simulink model "DDCU_wxt_v02_forA_LabviewV01"  (R2014a)
settings: Solver=FixedStepDiscrete  StartTime=0.0  StopTime=50  FixedStep=0.0005  RelTol=1e-3
InitFcn:
  | Veh_Par_wxt
values from neighbouring files (symbols this model uses):
  ag_thr = 0.4*g    (= 3.924)    [Veh_Par_wxt.m]
  B = 2.25    [Veh_Par_wxt.m]
  bra_pre_em = 12    [Veh_Par_wxt.m]
  bra_pre_gz2 = 12/3    (= 4)    [Veh_Par_wxt.m]
  bra_pre_gz34 = 12/3    (= 4)    [Veh_Par_wxt.m]
  bra_pre_yd = 12/2    (= 6)    [Veh_Par_wxt.m]
  brakepre_dem_data = [0 1 2 3 4 5 6 7 8 9 10 11 12]    [Veh_Par_wxt.m]
  brakeTrq_dem_data = [0 218.198 436.396 654.594 872.792 1090.99 1309.188 1527.386 1745.584 1963.782 2181.98 2400.178 2618.376]    [Veh_Par_wxt.m]
  bratrq_max = 4*2618.376    (= 10473.504)    [Veh_Par_wxt.m]
  eff_tran = 0.75    [Veh_Par_wxt.m]
  G = Mass*g    (= 36297)    [Veh_Par_wxt.m]
  kd1 = 1    [Veh_Par_wxt.m]
  kd2 = 1    [Veh_Par_wxt.m]
  kd3 = 1    [Veh_Par_wxt.m]
  ki1 = 1    [Veh_Par_wxt.m]
  ki2 = 1    [Veh_Par_wxt.m]
  ki3 = 1    [Veh_Par_wxt.m]
  kp1 = 1    [Veh_Par_wxt.m]
  kp2 = 1    [Veh_Par_wxt.m]
  kp3 = 1    [Veh_Par_wxt.m]
  L = 3.12    [Veh_Par_wxt.m]
  premax = 12    [Veh_Par_wxt.m]
  Radius = 0.20    (= 0.2)    [Veh_Par_wxt.m]
  s_opt_yi_add = 0.05    [Veh_Par_wxt.m]
  s_opt_zhuan_add = 0.05    [Veh_Par_wxt.m]
  spd_map_mot = [0 100 200 300 360 400 500 600 700 800 900]*tras_ratio    [Veh_Par_wxt.m]
  spdmax = 900*tras_ratio    (= 5580)    [Veh_Par_wxt.m]
  speed_thr_park = 5/3.6/Radius*30/pi    (= 66.3145596216)    [Veh_Par_wxt.m]
  tras_ratio = 6.2    [Veh_Par_wxt.m]
  trq_map_mot = [1200 1200 1200 1200 1200 1080 864 720 617 540 480]/tras_ratio    [Veh_Par_wxt.m]
  trqmax = 80    [Veh_Par_wxt.m]
  v_thr1_b = 5    [Veh_Par_wxt.m]
  v_thr2_b = 20    [Veh_Par_wxt.m]
  v_thr_park = 5    [Veh_Par_wxt.m]
undefined symbols (not defined in the file or in its folder): DiscIntNeverNeededParam
libraries: simulink x169, ec5744lib x9
(part 7 of 13)

== system DDCU_wxt_v02_forA_LabviewV01/MainControl/mode_control/forward/forward/Brake/rr ==
  speed_act_rr : Inport
  v_act : Inport  Port=2
  Add : Sum
  Constant : Constant  Value=eps
  Divide : Product  Inputs=*/
  Gain : Gain  Gain=pi/30
  Gain1 : Gain  Gain=Radius
  Gain2 : Gain  Gain=1/3.6
  Subtract : Sum  Inputs=+-
  s_act_rr : Outport
  wires:
  speed_act_rr/1 -> Gain/1
  Gain/1 -> Gain1/1
  v_act/1 -> Gain2/1
  Subtract/1 -> Divide/1
  Constant/1 -> Add/2
  Add/1 -> Divide/2
  Divide/1 -> s_act_rr/1
  Gain2/1 -> Add/1, Subtract/1
  Gain1/1 -> Subtract/2

== system DDCU_wxt_v02_forA_LabviewV01/MainControl/mode_control/forward/forward/Drive/容错控制 ==
  trq_dem_l : Inport
  trq_dem_r : Inport  Port=2
  trqlim_lf : Inport  Port=3
  trqlim_lr : Inport  Port=4
  trqlim_rf : Inport  Port=5
  trqlim_rr : Inport  Port=6
  guzhang_lf : Inport  Port=7
  guzhang_lr : Inport  Port=8
  guzhang_rf : Inport  Port=9
  guzhang_rr : Inport  Port=10
  Add : Sum
  Add1 : Sum
  Constant : Constant  Value=bra_pre_gz2
  Constant1 : Constant  Value=bra_pre_gz34
  MATLAB Function : MATLAB Function  TreatAsAtomicUnit=on
  Mux : Mux  Inputs=2
  Scope{,1..16} (17 alike) : Scope
      Scope settings: SaveName=ScopeData25
      Scope1 settings: SaveName=ScopeData26
      Scope10 settings: SaveName=ScopeData35
      Scope11 settings: SaveName=ScopeData36
      Scope12 settings: SaveName=ScopeData37
      Scope13 settings: SaveName=ScopeData38
      Scope14 settings: SaveName=ScopeData39
      Scope15 settings: SaveName=ScopeData40
      Scope16 settings: SaveName=ScopeData41
      Scope2 settings: SaveName=ScopeData27
      Scope3 settings: SaveName=ScopeData28
      Scope4 settings: SaveName=ScopeData29
      Scope5 settings: SaveName=ScopeData30
      Scope6 settings: SaveName=ScopeData31
      Scope7 settings: SaveName=ScopeData32
      Scope8 settings: SaveName=ScopeData33
      Scope9 settings: SaveName=ScopeData34
  Subtract : Sum  Inputs=+-
  To Workspace1 : ToWorkspace  VariableName=simout1  SaveFormat=Timeseries  SampleTime=-1
  To Workspace2 : ToWorkspace  VariableName=simout  SaveFormat=Timeseries  SampleTime=-1
  To Workspace3 : ToWorkspace  VariableName=simout2  SaveFormat=Timeseries  SampleTime=-1
  To Workspace4 : ToWorkspace  VariableName=simout3  SaveFormat=Timeseries  SampleTime=-1
  To Workspace5 : ToWorkspace  VariableName=simout4  SaveFormat=Timeseries  SampleTime=-1
  trq_dem_lf : Outport
  trq_dem_lr : Outport  Port=2
  trq_dem_rf : Outport  Port=3
  trq_dem_rr : Outport  Port=4
  bra_pre_l : Outport  Port=5
  bra_pre_r : Outport  Port=6
  wires:
  guzhang_lr/1 -> To Workspace3/1, MATLAB Function/8(guzhang_lr), Scope14/1
  guzhang_rf/1 -> Scope15/1, To Workspace4/1, MATLAB Function/9(guzhang_rf)
  guzhang_rr/1 -> Scope16/1, To Workspace5/1, MATLAB Function/10(guzhang_rr)
  guzhang_lf/1 -> To Workspace2/1, Scope13/1, MATLAB Function/7(guzhang_lf)
  trq_dem_r/1 -> Scope9/1, MATLAB Function/2(trq_dem_r)
  trqlim_lr/1 -> MATLAB Function/4(trqlim_lr)
  trq_dem_l/1 -> Scope8/1, MATLAB Function/1(trq_dem_l)
  trqlim_rf/1 -> Scope10/1, MATLAB Function/5(trqlim_rf)
  trqlim_rr/1 -> Scope12/1, MATLAB Function/6(trqlim_rr)
  trqlim_lf/1 -> MATLAB Function/3(trqlim_lf)
  MATLAB Function/1(trq_dem_lf) -> Scope/1, Add/1, trq_dem_lf/1
  MATLAB Function/2(trq_dem_lr) -> Scope1/1, Add/2, trq_dem_lr/1
  MATLAB Function/3(trq_dem_rf) -> Scope2/1, Add1/1, trq_dem_rf/1
  MATLAB Function/4(trq_dem_rr) -> Scope3/1, Add1/2, trq_dem_rr/1
  MATLAB Function/5(bra_pre_l) -> Scope4/1, bra_pre_l/1
  MATLAB Function/6(bra_pre_r) -> Scope5/1, bra_pre_r/1
  Constant/1 -> MATLAB Function/11(bra_pre_gz2)
  Constant1/1 -> MATLAB Function/12(bra_pre_gz34)
  Add/1 -> Mux/1, Subtract/1
  Add1/1 -> Mux/2, Subtract/2
  Subtract/1 -> Scope6/1
  Mux/1 -> Scope7/1
  MATLAB Function/7(mode) -> To Workspace1/1, Scope11/1

== system DDCU_wxt_v02_forA_LabviewV01/MainControl/mode_control/forward/forward/Drive/左右侧电机分配及功率限制 ==
  Trq_line_dem : Inport
  delta_T_dem : Inport  Port=2
  pwr_dis_bat : Inport  Port=3
  speed_act_lf : Inport  Port=4
  speed_act_lr : Inport  Port=5
  speed_act_rf : Inport  Port=6
  speed_act_rr : Inport  Port=7
  TrqLimU_dig_lf : Inport  Port=8
  TrqLimU_dig_lr : Inport  Port=9
  TrqLimU_dig_rf : Inport  Port=10
  TrqLimU_dig_rr : Inport  Port=11
  Add : Sum
  Add1 : Sum  Inputs=++++
  Add2 : Sum
  Add3 : Sum
  Constant : Constant  Value=9549
  Divide : Product  Inputs=**/
  Gain : Gain  Gain=1/4
  Gain1 : Gain  Gain=1/2
  Gain2 : Gain  Gain=1/2
  MATLAB Function : MATLAB Function  TreatAsAtomicUnit=on
  MinMax{,1..6} (7 alike) : MinMax  Inputs=2
  Mux : Mux  Inputs=2
  Scope{,1..10} (11 alike) : Scope
      Scope settings: SaveName=ScopeData14
      Scope1 settings: SaveName=ScopeData15
      Scope10 settings: SaveName=ScopeData24
      Scope2 settings: SaveName=ScopeData16
      Scope3 settings: SaveName=ScopeData17
      Scope4 settings: SaveName=ScopeData18
      Scope5 settings: SaveName=ScopeData19
      Scope6 settings: SaveName=ScopeData20
      Scope7 settings: SaveName=ScopeData21
      Scope8 settings: SaveName=ScopeData22
      Scope9 settings: SaveName=ScopeData23
  Subtract : Sum  Inputs=+-
  mot_map{,1..3} (4 alike) : Lookup_n-D  NumberOfTableDimensions=1  BreakpointsForDimension1=spd_map_mot  Table=trq_map_mot  InternalRulePriority=Speed  RndMeth=Simplest  InputSameDT=on
  trq_dem_l : Outport
  trq_dem_r : Outport  Port=2
  trqlim_lf : Outport  Port=3
  trqlim_lr : Outport  Port=4
  trqlim_rf : Outport  Port=5
  trqlim_rr : Outport  Port=6
  wires:
  speed_act_rf/1 -> mot_map2/1, Add1/3
  speed_act_lr/1 -> mot_map1/1, Add1/2
  speed_act_rr/1 -> mot_map3/1, Add1/4
  speed_act_lf/1 -> mot_map/1, Add1/1
  Add1/1 -> Gain/1
  Constant/1 -> Divide/1
  pwr_dis_bat/1 -> Divide/2
  Gain/1 -> Divide/3
  Divide/1 -> MinMax/1
  Trq_line_dem/1 -> MinMax/2
  MinMax/1 -> Gain1/1
  Gain1/1 -> Mux/1, Subtract/1, Add/1
  delta_T_dem/1 -> [delta_T_dem], Scope10/1, Gain2/1
  Subtract/1 -> Scope2/1, MinMax1/2
  MinMax1/1 -> Scope3/1, MATLAB Function/2(trq_dem_l1)
  Add/1 -> Scope8/1, MinMax2/2
  MinMax2/1 -> Scope7/1, MATLAB Function/4(trq_dem_r1)
  mot_map3/1 -> MinMax3/1
  TrqLimU_dig_rr/1 -> MinMax3/2
  mot_map2/1 -> MinMax4/1
  TrqLimU_dig_rf/1 -> MinMax4/2
  mot_map1/1 -> MinMax5/1
  TrqLimU_dig_lr/1 -> MinMax5/2
  mot_map/1 -> MinMax6/1
  TrqLimU_dig_lf/1 -> MinMax6/2
  MinMax6/1 -> trqlim_lf/1, Add3/1
  MinMax5/1 -> trqlim_lr/1, Add3/2
  MinMax4/1 -> trqlim_rf/1, Add2/1
  MinMax3/1 -> trqlim_rr/1, Add2/2
  Add3/1 -> [trqlim_l]
  [trqlim_l] -> Scope4/1, MATLAB Function/1(trqlim_l), MinMax1/1
  Add2/1 -> [trqlim_r]
  [trqlim_r] -> MATLAB Function/3(trqlim_r), MinMax2/1, Scope9/1
  [delta_T_dem] -> MATLAB Function/5(delta_T_dem)
  MATLAB Function/1(trq_dem_l) -> Scope/1, trq_dem_l/1
  MATLAB Function/2(trq_dem_r) -> Scope1/1, trq_dem_r/1
  Mux/1 -> Scope5/1
  Gain2/1 -> Scope6/1, Add/2, Subtract/2, Mux/2

== system DDCU_wxt_v02_forA_LabviewV01/MainControl/mode_control/forward/forward/Drive/目标直驶力矩确定模块 ==
  acc_dem : Inport
  v_act : Inport  Port=2
  TrqLimU_dig_lf : Inport  Port=3
  TrqLimU_dig_lr : Inport  Port=4
  TrqLimU_dig_rf : Inport  Port=5
  TrqLimU_dig_rr : Inport  Port=6
  Add : Sum  Inputs=++++
  Constant : Constant  Value=3.6
  Constant1 : Constant  Value=Radius
  Constant2 : Constant  Value=30/pi
  Divide : Product  Inputs=*//*
  Gain : Gain  Gain=1/100
  Gain1 : Gain  Gain=tras_ratio
  MinMax{,1..3} (4 alike) : MinMax  Inputs=2
  Product : Product
  Scope : Scope
      settings: SaveName=ScopeData7
  Scope1 : Scope
      settings: SaveName=ScopeData8
  mot_map : Lookup_n-D  NumberOfTableDimensions=1  BreakpointsForDimension1=spd_map_mot  Table=trq_map_mot  InternalRulePriority=Speed  RndMeth=Simplest  InputSameDT=on
  Trq_line_dem : Outport
  wires:
  Constant1/1 -> Divide/3
  Constant/1 -> Divide/2
  Constant2/1 -> Divide/4
  Divide/1 -> Gain1/1
  TrqLimU_dig_lf/1 -> MinMax/2
  mot_map/1 -> MinMax1/1, MinMax2/1, MinMax3/1, Scope1/1, MinMax/1
  TrqLimU_dig_lr/1 -> MinMax1/2
  TrqLimU_dig_rf/1 -> MinMax2/2
  TrqLimU_dig_rr/1 -> MinMax3/2
  MinMax1/1 -> Add/2
  MinMax2/1 -> Add/3
  MinMax/1 -> Add/1
  MinMax3/1 -> Add/4
  Add/1 -> Product/2
  acc_dem/1 -> Gain/1
  Product/1 -> Scope/1, Trq_line_dem/1
  Gain/1 -> Product/1
  Gain1/1 -> mot_map/1
  v_act/1 -> Divide/1

== system DDCU_wxt_v02_forA_LabviewV01/MainControl/mode_control/forward/forward/Drive/目标转向力矩确定模块 ==
  note: 左转为正，右转为负
  v_act : Inport
  TrqLimU_dig_lf : Inport  Port=2
  TrqLimU_dig_lr : Inport  Port=3
  TrqLimU_dig_rf : Inport  Port=4
  TrqLimU_dig_rr : Inport  Port=5
  steer_dem : Inport  Port=6
  umax : Inport  Port=7
  f : Inport  Port=8
  Action Port : ActionPort
  Add : Sum
  Add1 : Sum
  Constant : Constant  Value=3.6
  Constant1 : Constant  Value=Radius
  Constant2 : Constant  Value=30/pi
  Constant3 : Constant  Value=G
  Constant4 : Constant  Value=L
  Constant5 : Constant  Value=B
  Constant6 : Constant  Value=eff_tran
  Constant7 : Constant  Value=Radius
  Constant8 : Constant  Value=ag_thr
  Constant9 : Constant  Value=Radius
  Divide : Product  Inputs=*//*
  Gain : Gain  Gain=1/100
  Gain1 : Gain  Gain=tras_ratio
  Gain2 : Gain  Gain=tras_ratio
  Gain3 : Gain  Gain=1/tras_ratio
  Gain4 : Gain  Gain=tras_ratio
  MATLAB Function : MATLAB Function  TreatAsAtomicUnit=on
  MATLAB Function1 : MATLAB Function  TreatAsAtomicUnit=on
  MATLAB Function2 : MATLAB Function  TreatAsAtomicUnit=on
  MinMax{,1..3} (4 alike) : MinMax  Inputs=2
  MinMax4 : MinMax  Function=max  Inputs=2
  Product : Product
  Scope{,1..3} (4 alike) : Scope
      Scope settings: SaveName=ScopeData10
      Scope1 settings: SaveName=ScopeData11
      Scope2 settings: SaveName=ScopeData12
      Scope3 settings: SaveName=ScopeData13
  mot_map : Lookup_n-D  NumberOfTableDimensions=1  BreakpointsForDimension1=spd_map_mot  Table=trq_map_mot  InternalRulePriority=Speed  RndMeth=Simplest  InputSameDT=on
  delta_Tsteer_dem : Outport
  wires:
  Gain/1 -> Product/1
  Product/1 -> Gain3/1, Scope3/1
  [steer_dem] -> Gain/1
  MinMax3/1 -> Add1/2
  MinMax/1 -> Add/1
  MinMax2/1 -> Add1/1
  MinMax1/1 -> Add/2
  TrqLimU_dig_rr/1 -> MinMax3/2
  TrqLimU_dig_rf/1 -> MinMax2/2
  TrqLimU_dig_lr/1 -> MinMax1/2
  mot_map/1 -> MinMax/1, MinMax3/1, MinMax2/1, MinMax1/1
  TrqLimU_dig_lf/1 -> MinMax/2
  Divide/1 -> Gain1/1
  Constant2/1 -> Divide/4
  Constant/1 -> Divide/2
  Constant1/1 -> Divide/3
  steer_dem/1 -> [steer_dem], MATLAB Function/1(steer_dem)
  Constant3/1 -> [G], MATLAB Function/2(G)
  Constant4/1 -> [L], MATLAB Function/3(L)
  Constant5/1 -> [B], MATLAB Function/5(B)
  umax/1 -> [umax], MATLAB Function/4(umax)
  Add/1 -> Gain2/1
  Add1/1 -> Gain4/1
  Constant6/1 -> MATLAB Function/8(eff_tran)
  Constant7/1 -> MATLAB Function/9(Radius)
  f/1 -> MATLAB Function/10(f)
  MATLAB Function/1(Rturn_min) -> Scope/1, MinMax4/1
  [v_act] -> MATLAB Function1/1(v_act)
  Constant8/1 -> MATLAB Function1/2(ag_thr)
  MATLAB Function1/1(Rturn_min_ag) -> MinMax4/2, Scope1/1
  [umax] -> MATLAB Function2/1(umax)
  [G] -> MATLAB Function2/2(G)
  [L] -> MATLAB Function2/3(L)
  [B] -> MATLAB Function2/4(B)
  Constant9/1 -> MATLAB Function2/5(Radius)
  MinMax4/1 -> MATLAB Function2/6(Rturn_min_xy)
  MATLAB Function2/1(delta_Tsteer_max) -> Scope2/1, Product/2
  Gain1/1 -> mot_map/1
  v_act/1 -> Divide/1, [v_act]
  Gain3/1 -> delta_Tsteer_dem/1
  Gain2/1 -> MATLAB Function/6(Tpeak_L)
  Gain4/1 -> MATLAB Function/7(Tpeak_R)

== system DDCU_wxt_v02_forA_LabviewV01/MainControl/mode_control/forward/forward/Drive/直驶纠偏控制 ==
  dis_east : Inport
  dis_north : Inport  Port=2
  hangxiangangle : Inport  Port=3
  Action Port : ActionPort
  Constant : Constant  Value=0
  Terminator : Terminator
  Terminator1 : Terminator
  Terminator2 : Terminator
  delta_Tjiupian : Outport
  wires:
  Constant/1 -> delta_Tjiupian/1
  dis_east/1 -> Terminator/1
  dis_north/1 -> Terminator1/1
  hangxiangangle/1 -> Terminator2/1

== system DDCU_wxt_v02_forA_LabviewV01/MainControl/mode_control/forward/forward/Drive/路面状况识别模块 ==
  In1 : Inport
  Constant : Constant  Value=0.9
  Constant1 : Constant  Value=0.05
  Constant2 : Constant  Value=0.15
  Constant3 : Constant  Value=0.15
  Terminator : Terminator
  umax : Outport
  f : Outport  Port=2
  s_opt_zhuan : Outport  Port=3
  s_opt_yi : Outport  Port=4
  wires:
  Constant/1 -> umax/1
  Constant1/1 -> f/1
  Constant2/1 -> s_opt_zhuan/1
  Constant3/1 -> s_opt_yi/1
  In1/1 -> Terminator/1

== system DDCU_wxt_v02_forA_LabviewV01/MainControl/mode_control/forward/forward/Drive/车辆稳定性控制 ==
  note: 加速度向左为正
  acc_y : Inport
  Action Port : ActionPort
  Abs : Abs
  Add : Sum  Inputs=+++
  Constant : Constant  Value=ag_thr
  Constant1 : Constant
  Constant2 : Constant  Value=-1
  Difference : simulink/Discrete/Difference  ICPrevInput=0.0  InputProcessing=Inherited  OutMin=[]  OutMax=[]  OutDataType=fixdt(1, 16)  OutScaling=2^-10  DoSatur=off
  Discrete-Time Integrator : DiscreteIntegrator  SampleTime=-1  ICPrevOutput=DiscIntNeverNeededParam  ICPrevScaledInput=DiscIntNeverNeededParam
  Gain : Gain  Gain=kp1
  Gain1 : Gain  Gain=ki1
  Gain2 : Gain  Gain=kd1
  Gain3 : Gain  Gain=1/tras_ratio
  Product : Product
  Sum : Sum  Inputs=|+-
  Switch : Switch
  delta_Twending_dem : Outport
  wires:
  Constant/1 -> Sum/1
  acc_y/1 -> Switch/2, Abs/1
  Gain/1 -> Add/1
  Gain1/1 -> Discrete-Time Integrator/1
  Gain2/1 -> Difference/1
  Abs/1 -> Sum/2
  Constant1/1 -> Switch/1
  Constant2/1 -> Switch/3
  Switch/1 -> Product/2
  Product/1 -> Gain3/1
  Add/1 -> Product/1
  Sum/1 -> Gain2/1, Gain1/1, Gain/1
  Discrete-Time Integrator/1 -> Add/2
  Difference/1 -> Add/3
  Gain3/1 -> delta_Twending_dem/1

== system DDCU_wxt_v02_forA_LabviewV01/MainControl/mode_control/forward/forward/Drive/驱动防滑控制TCS ==
  trq_dem_lf : Inport
  trq_dem_lr : Inport  Port=2
  trq_dem_rf : Inport  Port=3
  trq_dem_rr : Inport  Port=4
  bra_pre_l : Inport  Port=5
  bra_pre_r : Inport  Port=6
  speed_act_lf : Inport  Port=7
  speed_act_lr : Inport  Port=8
  speed_act_rf : Inport  Port=9
  speed_act_rr : Inport  Port=10
  v_act : Inport  Port=11
  steer_dem : Inport  Port=12
  acc_y : Inport  Port=13
  brake_dem : Inport  Port=14
  s_opt_zhuan : Inport  Port=15
  MATLAB Function : MATLAB Function  TreatAsAtomicUnit=on
  Multiport Switch : MultiPortSwitch  DataPortOrder=Zero-based contiguous  Inputs=2
  Switch Case : SwitchCase  CaseConditions={0,1}  ShowDefaultCase=off
  直行TCS : Subsystem  TreatAsAtomicUnit=on
  转向TCS : Subsystem  TreatAsAtomicUnit=on
  forward_dem : Outport
  wires:
  steer_dem/1 -> 转向TCS/1(steer_dem), 直行TCS/1(steer_dem), MATLAB Function/1(steer_dem)
  MATLAB Function/1(y) -> Multiport Switch/1, Switch Case/1
  Switch Case/1 -> 转向TCS/Action
  Switch Case/2 -> 直行TCS/Action
  trq_dem_lf/1 -> 直行TCS/2(trq_dem_lf), 转向TCS/2(trq_dem_lf)
  trq_dem_lr/1 -> 直行TCS/3(trq_dem_lr), 转向TCS/3(trq_dem_lr)
  trq_dem_rf/1 -> 直行TCS/4(trq_dem_rf), 转向TCS/4(trq_dem_rf)
  trq_dem_rr/1 -> 直行TCS/5(trq_dem_rr), 转向TCS/5(trq_dem_rr)
  bra_pre_l/1 -> 直行TCS/6(bra_pre_l), 转向TCS/6(bra_pre_l)
  bra_pre_r/1 -> 直行TCS/7(bra_pre_r), 转向TCS/7(bra_pre_r)
  speed_act_lf/1 -> 直行TCS/8(speed_act_lf), 转向TCS/8(speed_act_lf)
  speed_act_lr/1 -> 直行TCS/9(speed_act_lr), 转向TCS/9(speed_act_lr)
  speed_act_rf/1 -> 直行TCS/10(speed_act_rf), 转向TCS/10(speed_act_rf)
  speed_act_rr/1 -> 直行TCS/11(speed_act_rr), 转向TCS/11(speed_act_rr)
  v_act/1 -> 直行TCS/12(v_act), 转向TCS/12(v_act)
  acc_y/1 -> 直行TCS/13(acc_y), 转向TCS/13(acc_y)
  s_opt_zhuan/1 -> 直行TCS/15(s_opt_zhuan), 转向TCS/15(s_opt_zhuan)
  brake_dem/1 -> 直行TCS/14(brake_dem), 转向TCS/14(brake_dem)
  直行TCS/1(forward_dem) -> Multiport Switch/3
  转向TCS/1(forward_dem) -> Multiport Switch/2
  Multiport Switch/1 -> forward_dem/1

== system DDCU_wxt_v02_forA_LabviewV01/MainControl/mode_control/backward/backward/Drive/驱动防滑控制TCS/直行TCS ==
  steer_dem : Inport
  trq_dem_lf : Inport  Port=2
  trq_dem_lr : Inport  Port=3
  trq_dem_rf : Inport  Port=4
  trq_dem_rr : Inport  Port=5
  bra_pre_l : Inport  Port=6
  bra_pre_r : Inport  Port=7
  speed_act_lf : Inport  Port=8
  speed_act_lr : Inport  Port=9
  speed_act_rf : Inport  Port=10
  speed_act_rr : Inport  Port=11
  v_act : Inport  Port=12
  acc_y : Inport  Port=13
  brake_dem : Inport  Port=14
  s_opt_zhuan : Inport  Port=15
  Action Port : ActionPort
  Scope : Scope  NumInputPorts=4
      settings: YMin=-5~-5~-5~-5  YMax=5~5~5~5  SaveName=ScopeData42
  Subsystem : Subsystem
  Subsystem1 : Subsystem
  Subsystem2 : Subsystem
  Subsystem3 : Subsystem
  Terminator : Terminator
  Terminator1 : Terminator
  直行 : Subsystem  TreatAsAtomicUnit=on
  backward_dem : Outport
  wires:
  steer_dem/1 -> Terminator1/1
  speed_act_lf/1 -> Subsystem/1(speed_act_lf)
  v_act/1 -> Subsystem2/2(v_act), Subsystem1/2(v_act), Subsystem/2(v_act), Subsystem3/2(v_act)
  speed_act_lr/1 -> Subsystem1/1(speed_act_lr)
  speed_act_rf/1 -> Subsystem2/1(speed_act_rf)
  speed_act_rr/1 -> Subsystem3/1(speed_act_rr)
  acc_y/1 -> Terminator/1
  trq_dem_lr/1 -> 直行/2(trq_dem_lr)
  trq_dem_lf/1 -> 直行/1(trq_dem_lf)
  trq_dem_rf/1 -> 直行/3(trq_dem_rf)
  trq_dem_rr/1 -> 直行/4(trq_dem_rr)
  bra_pre_l/1 -> 直行/5(bra_pre_l)
  bra_pre_r/1 -> 直行/6(bra_pre_r)
  Subsystem/1(s_act_lf) -> 直行/7(s_act_lf), Scope/1
  Subsystem1/1(s_act_lr) -> 直行/8(s_act_lr), Scope/2
  Subsystem2/1(s_act_rf) -> 直行/9(s_act_rf), Scope/3
  Subsystem3/1(s_act_rr) -> 直行/10(s_act_rr), Scope/4
  s_opt_zhuan/1 -> 直行/12(s_opt_zhuan)
  brake_dem/1 -> 直行/11(brake_dem)
  直行/1(backward_dem) -> backward_dem/1

== system DDCU_wxt_v02_forA_LabviewV01/MainControl/mode_control/backward/backward/Drive/驱动防滑控制TCS/转向TCS ==
  steer_dem : Inport
  trq_dem_lf : Inport  Port=2
  trq_dem_lr : Inport  Port=3
  trq_dem_rf : Inport  Port=4
  trq_dem_rr : Inport  Port=5
  bra_pre_l : Inport  Port=6
  bra_pre_r : Inport  Port=7
  speed_act_lf : Inport  Port=8
  speed_act_lr : Inport  Port=9
  speed_act_rf : Inport  Port=10
  speed_act_rr : Inport  Port=11
  v_act : Inport  Port=12
  acc_y : Inport  Port=13
  brake_dem : Inport  Port=14
  s_opt_zhuan : Inport  Port=15
  Action Port : ActionPort
  MATLAB Function : MATLAB Function  TreatAsAtomicUnit=on
  Multiport Switch : MultiPortSwitch  DataPortOrder=Zero-based contiguous  Inputs=2
  Subsystem : Subsystem
  Subsystem1 : Subsystem
  Subsystem2 : Subsystem
  Subsystem3 : Subsystem
  Switch Case : SwitchCase  CaseConditions={0,1}  ShowDefaultCase=off
  Terminator : Terminator
  右转 : Subsystem  TreatAsAtomicUnit=on
  左转 : Subsystem  TreatAsAtomicUnit=on
  backward_dem : Outport
  wires:
  Multiport Switch/1 -> backward_dem/1
  右转/1(backward_dem) -> Multiport Switch/3
  左转/1(backward_dem) -> Multiport Switch/2
  brake_dem/1 -> 左转/11(brake_dem), 右转/11(brake_dem)
  s_opt_zhuan/1 -> 左转/12(s_opt_zhuan), 右转/12(s_opt_zhuan)
  Subsystem3/1(s_act_rr) -> 左转/10(s_act_rr), 右转/10(s_act_rr)
  Subsystem2/1(s_act_rf) -> 左转/9(s_act_rf), 右转/9(s_act_rf)
  Subsystem1/1(s_act_lr) -> 左转/8(s_act_lr), 右转/8(s_act_lr)
  Subsystem/1(s_act_lf) -> 左转/7(s_act_lf), 右转/7(s_act_lf)
  bra_pre_r/1 -> 左转/6(bra_pre_r), 右转/6(bra_pre_r)
  bra_pre_l/1 -> 左转/5(bra_pre_l), 右转/5(bra_pre_l)
  trq_dem_rr/1 -> 左转/4(trq_dem_rr), 右转/4(trq_dem_rr)
  trq_dem_rf/1 -> 左转/3(trq_dem_rf), 右转/3(trq_dem_rf)
  trq_dem_lf/1 -> 左转/1(trq_dem_lf), 右转/1(trq_dem_lf)
  trq_dem_lr/1 -> 左转/2(trq_dem_lr), 右转/2(trq_dem_lr)
  acc_y/1 -> Terminator/1
  Switch Case/2 -> 右转/Action
  Switch Case/1 -> 左转/Action
  speed_act_rr/1 -> Subsystem3/1(speed_act_rr)
  speed_act_rf/1 -> Subsystem2/1(speed_act_rf)
  speed_act_lr/1 -> Subsystem1/1(speed_act_lr)
  v_act/1 -> Subsystem3/2(v_act), Subsystem/2(v_act), Subsystem1/2(v_act), Subsystem2/2(v_act)
  speed_act_lf/1 -> Subsystem/1(speed_act_lf)
  MATLAB Function/1(y) -> Switch Case/1, Multiport Switch/1
  steer_dem/1 -> MATLAB Function/1(steer_dem)

== system DDCU_wxt_v02_forA_LabviewV01/MainControl/mode_control/forward/forward/Drive/驱动防滑控制TCS/直行TCS ==
  steer_dem : Inport
  trq_dem_lf : Inport  Port=2
  trq_dem_lr : Inport  Port=3
  trq_dem_rf : Inport  Port=4
  trq_dem_rr : Inport  Port=5
  bra_pre_l : Inport  Port=6
  bra_pre_r : Inport  Port=7
  speed_act_lf : Inport  Port=8
  speed_act_lr : Inport  Port=9
  speed_act_rf : Inport  Port=10
  speed_act_rr : Inport  Port=11
  v_act : Inport  Port=12
  acc_y : Inport  Port=13
  brake_dem : Inport  Port=14
  s_opt_zhuan : Inport  Port=15
  Action Port : ActionPort
  Scope : Scope  NumInputPorts=4
      settings: YMin=-5~-5~-5~-5  YMax=5~5~5~5  SaveName=ScopeData42
  Subsystem : Subsystem
  Subsystem1 : Subsystem
  Subsystem2 : Subsystem
  Subsystem3 : Subsystem
  Terminator : Terminator
  Terminator1 : Terminator
  直行 : Subsystem  TreatAsAtomicUnit=on
  forward_dem : Outport
  wires:
  直行/1(forward_dem) -> forward_dem/1
  brake_dem/1 -> 直行/11(brake_dem)
  s_opt_zhuan/1 -> 直行/12(s_opt_zhuan)
  Subsystem3/1(s_act_rr) -> Scope/4, 直行/10(s_act_rr)
  Subsystem2/1(s_act_rf) -> Scope/3, 直行/9(s_act_rf)
  Subsystem1/1(s_act_lr) -> Scope/2, 直行/8(s_act_lr)
  Subsystem/1(s_act_lf) -> Scope/1, 直行/7(s_act_lf)
  bra_pre_r/1 -> 直行/6(bra_pre_r)
  bra_pre_l/1 -> 直行/5(bra_pre_l)
  trq_dem_rr/1 -> 直行/4(trq_dem_rr)
  trq_dem_rf/1 -> 直行/3(trq_dem_rf)
  trq_dem_lf/1 -> 直行/1(trq_dem_lf)
  trq_dem_lr/1 -> 直行/2(trq_dem_lr)
  acc_y/1 -> Terminator/1
  speed_act_rr/1 -> Subsystem3/1(speed_act_rr)
  speed_act_rf/1 -> Subsystem2/1(speed_act_rf)
  speed_act_lr/1 -> Subsystem1/1(speed_act_lr)
  v_act/1 -> Subsystem3/2(v_act), Subsystem/2(v_act), Subsystem1/2(v_act), Subsystem2/2(v_act)
  speed_act_lf/1 -> Subsystem/1(speed_act_lf)
  steer_dem/1 -> Terminator1/1

== system DDCU_wxt_v02_forA_LabviewV01/MainControl/mode_control/forward/forward/Drive/驱动防滑控制TCS/转向TCS ==
  steer_dem : Inport
  trq_dem_lf : Inport  Port=2
  trq_dem_lr : Inport  Port=3
  trq_dem_rf : Inport  Port=4
  trq_dem_rr : Inport  Port=5
  bra_pre_l : Inport  Port=6
  bra_pre_r : Inport  Port=7
  speed_act_lf : Inport  Port=8
  speed_act_lr : Inport  Port=9
  speed_act_rf : Inport  Port=10
  speed_act_rr : Inport  Port=11
  v_act : Inport  Port=12
  acc_y : Inport  Port=13
  brake_dem : Inport  Port=14
  s_opt_zhuan : Inport  Port=15
  Action Port : ActionPort
  MATLAB Function : MATLAB Function  TreatAsAtomicUnit=on
  Multiport Switch : MultiPortSwitch  DataPortOrder=Zero-based contiguous  Inputs=2
  Subsystem : Subsystem
  Subsystem1 : Subsystem
  Subsystem2 : Subsystem
  Subsystem3 : Subsystem
  Switch Case : SwitchCase  CaseConditions={0,1}  ShowDefaultCase=off
  Terminator : Terminator
  右转 : Subsystem  TreatAsAtomicUnit=on
  左转 : Subsystem  TreatAsAtomicUnit=on
  forward_dem : Outport
  wires:
  steer_dem/1 -> MATLAB Function/1(steer_dem)
  MATLAB Function/1(y) -> Multiport Switch/1, Switch Case/1
  speed_act_lf/1 -> Subsystem/1(speed_act_lf)
  v_act/1 -> Subsystem2/2(v_act), Subsystem1/2(v_act), Subsystem/2(v_act), Subsystem3/2(v_act)
  speed_act_lr/1 -> Subsystem1/1(speed_act_lr)
  speed_act_rf/1 -> Subsystem2/1(speed_act_rf)
  speed_act_rr/1 -> Subsystem3/1(speed_act_rr)
  Switch Case/1 -> 左转/Action
  Switch Case/2 -> 右转/Action
  acc_y/1 -> Terminator/1
  trq_dem_lr/1 -> 右转/2(trq_dem_lr), 左转/2(trq_dem_lr)
  trq_dem_lf/1 -> 右转/1(trq_dem_lf), 左转/1(trq_dem_lf)
  trq_dem_rf/1 -> 右转/3(trq_dem_rf), 左转/3(trq_dem_rf)
  trq_dem_rr/1 -> 右转/4(trq_dem_rr), 左转/4(trq_dem_rr)
  bra_pre_l/1 -> 右转/5(bra_pre_l), 左转/5(bra_pre_l)
  bra_pre_r/1 -> 右转/6(bra_pre_r), 左转/6(bra_pre_r)
  Subsystem/1(s_act_lf) -> 右转/7(s_act_lf), 左转/7(s_act_lf)
  Subsystem1/1(s_act_lr) -> 右转/8(s_act_lr), 左转/8(s_act_lr)
  Subsystem2/1(s_act_rf) -> 右转/9(s_act_rf), 左转/9(s_act_rf)
  Subsystem3/1(s_act_rr) -> 右转/10(s_act_rr), 左转/10(s_act_rr)
  s_opt_zhuan/1 -> 右转/12(s_opt_zhuan), 左转/12(s_opt_zhuan)
  brake_dem/1 -> 右转/11(brake_dem), 左转/11(brake_dem)
  左转/1(forward_dem) -> Multiport Switch/2
  右转/1(forward_dem) -> Multiport Switch/3
  Multiport Switch/1 -> forward_dem/1

== system DDCU_wxt_v02_forA_LabviewV01/MainControl/mode_control/backward/backward/Drive/驱动防滑控制TCS/直行TCS/Subsystem ==
  speed_act_lf : Inport
  v_act : Inport  Port=2
  Add : Sum
  Constant : Constant  Value=eps
  Divide : Product  Inputs=*/
  Gain : Gain  Gain=pi/30
  Gain1 : Gain  Gain=Radius
  Gain2 : Gain  Gain=1/3.6
  Subtract : Sum  Inputs=+-
  s_act_lf : Outport
  wires:
  speed_act_lf/1 -> Gain/1
  Gain/1 -> Gain1/1
  v_act/1 -> Gain2/1
  Gain1/1 -> Add/1, Subtract/1
  Gain2/1 -> Subtract/2
  Subtract/1 -> Divide/1
  Constant/1 -> Add/2
  Add/1 -> Divide/2
  Divide/1 -> s_act_lf/1

== system DDCU_wxt_v02_forA_LabviewV01/MainControl/mode_control/backward/backward/Drive/驱动防滑控制TCS/直行TCS/Subsystem1 ==
  speed_act_lr : Inport
  v_act : Inport  Port=2
  Add : Sum
  Constant : Constant  Value=eps
  Divide : Product  Inputs=*/
  Gain : Gain  Gain=pi/30
  Gain1 : Gain  Gain=Radius
  Gain2 : Gain  Gain=1/3.6
  Subtract : Sum  Inputs=+-
  s_act_lr : Outport
  wires:
  Divide/1 -> s_act_lr/1
  Add/1 -> Divide/2
  Constant/1 -> Add/2
  Subtract/1 -> Divide/1
  Gain2/1 -> Subtract/2
  Gain1/1 -> Subtract/1, Add/1
  v_act/1 -> Gain2/1
  Gain/1 -> Gain1/1
  speed_act_lr/1 -> Gain/1

== system DDCU_wxt_v02_forA_LabviewV01/MainControl/mode_control/backward/backward/Drive/驱动防滑控制TCS/直行TCS/Subsystem2 ==
  speed_act_rf : Inport
  v_act : Inport  Port=2
  Add : Sum
  Constant : Constant  Value=eps
  Divide : Product  Inputs=*/
  Gain : Gain  Gain=pi/30
  Gain1 : Gain  Gain=Radius
  Gain2 : Gain  Gain=1/3.6
  Subtract : Sum  Inputs=+-
  s_act_rf : Outport
  wires:
  speed_act_rf/1 -> Gain/1
  Gain/1 -> Gain1/1
  v_act/1 -> Gain2/1
  Gain1/1 -> Add/1, Subtract/1
  Gain2/1 -> Subtract/2
  Subtract/1 -> Divide/1
  Constant/1 -> Add/2
  Add/1 -> Divide/2
  Divide/1 -> s_act_rf/1

== system DDCU_wxt_v02_forA_LabviewV01/MainControl/mode_control/backward/backward/Drive/驱动防滑控制TCS/直行TCS/Subsystem3 ==
  speed_act_rr : Inport
  v_act : Inport  Port=2
  Add : Sum
  Constant : Constant  Value=eps
  Divide : Product  Inputs=*/
  Gain : Gain  Gain=pi/30
  Gain1 : Gain  Gain=Radius
  Gain2 : Gain  Gain=1/3.6
  Subtract : Sum  Inputs=+-
  s_act_rr : Outport
  wires:
  Divide/1 -> s_act_rr/1
  Add/1 -> Divide/2
  Constant/1 -> Add/2
  Subtract/1 -> Divide/1
  Gain2/1 -> Subtract/2
  Gain1/1 -> Subtract/1, Add/1
  v_act/1 -> Gain2/1
  Gain/1 -> Gain1/1
  speed_act_rr/1 -> Gain/1

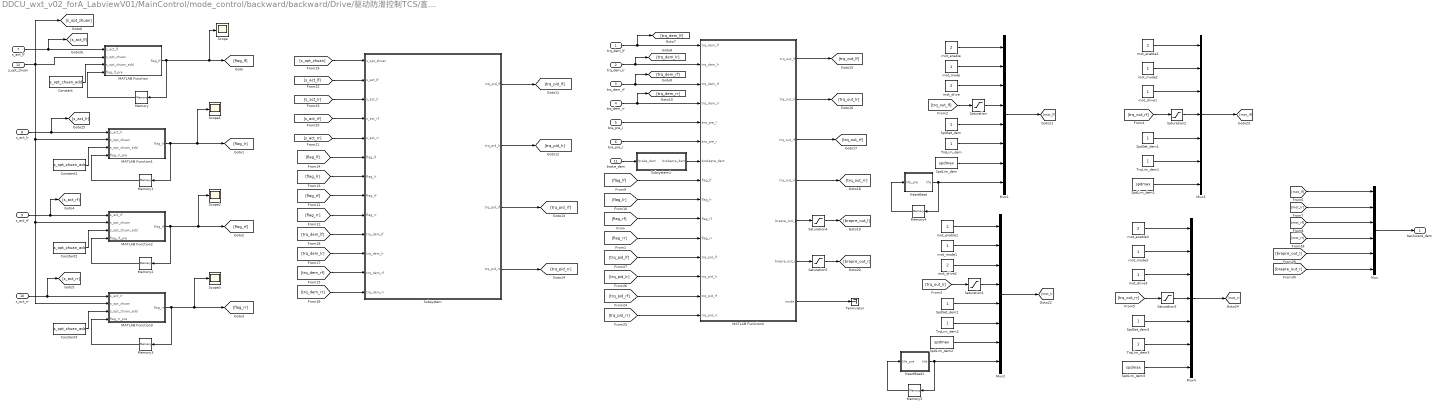
== system DDCU_wxt_v02_forA_LabviewV01/MainControl/mode_control/backward/backward/Drive/驱动防滑控制TCS/直行TCS/直行 ==
  trq_dem_lf : Inport
  trq_dem_lr : Inport  Port=2
  trq_dem_rf : Inport  Port=3
  trq_dem_rr : Inport  Port=4
  bra_pre_l : Inport  Port=5
  bra_pre_r : Inport  Port=6
  s_act_lf : Inport  Port=7
  s_act_lr : Inport  Port=8
  s_act_rf : Inport  Port=9
  s_act_rr : Inport  Port=10
  brake_dem : Inport  Port=11
  s_opt_zhuan : Inport  Port=12
  Constant{,1..3} (4 alike) : Constant  Value=s_opt_zhuan_add
  HeartBeat : MATLAB Function  TreatAsAtomicUnit=on
  HeartBeat1 : MATLAB Function  TreatAsAtomicUnit=on
  MATLAB Function : MATLAB Function  TreatAsAtomicUnit=on
  MATLAB Function1 : MATLAB Function  TreatAsAtomicUnit=on
  MATLAB Function2 : MATLAB Function  TreatAsAtomicUnit=on
  MATLAB Function3 : MATLAB Function  TreatAsAtomicUnit=on
  MATLAB Function4 : MATLAB Function  TreatAsAtomicUnit=on
  Memory{,1..5} (6 alike) : Memory  InheritSampleTime=on
  Mux : Mux  Inputs=6
  Mux1 : Mux  Inputs=8
  Mux2 : Mux  Inputs=8
  Mux3 : Mux  Inputs=7
  Mux4 : Mux  Inputs=7
  Saturation{,1..3} (4 alike) : Saturate  UpperLimit=trqmax  LowerLimit=0
  Saturation4 : Saturate  UpperLimit=premax  LowerLimit=0
  Saturation5 : Saturate  UpperLimit=premax  LowerLimit=0
  Scope{,1..3} (4 alike) : Scope
      Scope settings: SaveName=ScopeData43
      Scope1 settings: SaveName=ScopeData44
      Scope2 settings: SaveName=ScopeData45
      Scope3 settings: SaveName=ScopeData46
  SpdLim_dem{,1..3} (4 alike) : Constant  Value=spdmax
  SpdSet_dem{,1..3} (4 alike) : Constant
  Subsystem : Subsystem
  Subsystem1 : Subsystem
  Terminator : Terminator
  TrqLim_dem{,1..3} (4 alike) : Constant
  mot_drive : Constant  Value=2
  mot_drive1 : Constant
  mot_drive2 : Constant  Value=2
  mot_drive3 : Constant
  mot_enable{,1..3} (4 alike) : Constant  Value=2
  mot_mode{,1..3} (4 alike) : Constant
  backward_dem : Outport
  wires:
  Saturation5/1 -> [brapre_out_r]
  Saturation4/1 -> [brapre_out_l]
  Saturation3/1 -> Mux4/4
  Saturation1/1 -> Mux2/4
  Saturation2/1 -> Mux3/4
  Saturation/1 -> Mux1/4
  MATLAB Function4/7(mode) -> Terminator/1
  brake_dem/1 -> Subsystem1/1(brake_dem)
  Subsystem1/1(brakepre_dem) -> MATLAB Function4/7(brakepre_dem)
  [brapre_out_r] -> Mux/6
  [brapre_out_l] -> Mux/5
  [mot_rr] -> Mux/4
  [mot_rf] -> Mux/3
  [mot_lr] -> Mux/2
  [mot_lf] -> Mux/1
  MATLAB Function4/6(brapre_out_r) -> Saturation5/1
  MATLAB Function4/5(brapre_out_l) -> Saturation4/1
  MATLAB Function4/4(trq_out_rr) -> [trq_out_rr]
  MATLAB Function4/3(trq_out_rf) -> [trq_out_rf]
  MATLAB Function4/2(trq_out_lr) -> [trq_out_lr]
  MATLAB Function4/1(trq_out_lf) -> [trq_out_lf]
  mot_drive/1 -> Mux1/3
  mot_mode/1 -> Mux1/2
  [trq_out_lf] -> Saturation/1
  mot_enable/1 -> Mux1/1
  SpdSet_dem/1 -> Mux1/5
  Mux1/1 -> [mot_lf]
  TrqLim_dem/1 -> Mux1/6
  HeartBeat/1(life) -> Mux1/8, Memory4/1
  Memory4/1 -> HeartBeat/1(life_pre)
  SpdLim_dem/1 -> Mux1/7
  mot_drive1/1 -> Mux3/3
  mot_mode2/1 -> Mux3/2
  [trq_out_rf] -> Saturation2/1
  mot_enable2/1 -> Mux3/1
  SpdSet_dem1/1 -> Mux3/5
  Mux3/1 -> [mot_rf]
  TrqLim_dem1/1 -> Mux3/6
  SpdLim_dem1/1 -> Mux3/7
  mot_drive2/1 -> Mux2/3
  mot_mode1/1 -> Mux2/2
  [trq_out_lr] -> Saturation1/1
  mot_enable1/1 -> Mux2/1
  SpdSet_dem2/1 -> Mux2/5
  Mux2/1 -> [mot_lr]
  TrqLim_dem2/1 -> Mux2/6
  HeartBeat1/1(life) -> Mux2/8, Memory5/1
  Memory5/1 -> HeartBeat1/1(life_pre)
  SpdLim_dem2/1 -> Mux2/7
  mot_drive3/1 -> Mux4/3
  mot_mode3/1 -> Mux4/2
  [trq_out_rr] -> Saturation3/1
  mot_enable3/1 -> Mux4/1
  SpdSet_dem3/1 -> Mux4/5
  Mux4/1 -> [mot_rr]
  TrqLim_dem3/1 -> Mux4/6
  SpdLim_dem3/1 -> Mux4/7
  bra_pre_r/1 -> MATLAB Function4/6(bra_pre_r)
  bra_pre_l/1 -> MATLAB Function4/5(bra_pre_l)
  trq_dem_rr/1 -> [trq_dem_rr], MATLAB Function4/4(trq_dem_rr)
  trq_dem_rf/1 -> [trq_dem_rf], MATLAB Function4/3(trq_dem_rf)
  trq_dem_lr/1 -> [trq_dem_lr], MATLAB Function4/2(trq_dem_lr)
  trq_dem_lf/1 -> [trq_dem_lf], MATLAB Function4/1(trq_dem_lf)
  [trq_pid_rr] -> MATLAB Function4/15(trq_pid_rr)
  [trq_pid_rf] -> MATLAB Function4/14(trq_pid_rf)
  [trq_pid_lr] -> MATLAB Function4/13(trq_pid_lr)
  [trq_pid_lf] -> MATLAB Function4/12(trq_pid_lf)
  Subsystem/3(trq_pid_rf) -> [trq_pid_rf]
  Subsystem/4(trq_pid_rr) -> [trq_pid_rr]
  Subsystem/1(trq_pid_lf) -> [trq_pid_lf]
  Subsystem/2(trq_pid_lr) -> [trq_pid_lr]
  [s_act_lf] -> Subsystem/2(s_act_lf)
  [s_act_lr] -> Subsystem/3(s_act_lr)
  [s_act_rf] -> Subsystem/4(s_act_rf)
  [s_act_rr] -> Subsystem/5(s_act_rr)
  [s_opt_zhuan] -> Subsystem/1(s_opt_zhuan)
  [flag_rr] -> Subsystem/9(flag_rr)
  [trq_dem_rr] -> Subsystem/13(trq_dem_rr)
  [flag_rf] -> Subsystem/8(flag_rf)
  [flag_lr] -> Subsystem/7(flag_lr)
  [trq_dem_lr] -> Subsystem/11(trq_dem_lr)
  [trq_dem_rf] -> Subsystem/12(trq_dem_rf)
  [flag_lf] -> Subsystem/6(flag_lf)
  [trq_dem_lf] -> Subsystem/10(trq_dem_lf)
  [flag_lf] -> MATLAB Function4/8(flag_lf)
  [flag_lr] -> MATLAB Function4/9(flag_lr)
  s_act_lf/1 -> MATLAB Function/1(s_act_lf), [s_act_lf]
  MATLAB Function/1(flag_lf) -> Memory/1, [flag_lf], Scope/1
  Memory/1 -> MATLAB Function/4(flag_lf_pre)
  Constant/1 -> MATLAB Function/3(s_opt_zhuan_add)
  s_act_lr/1 -> MATLAB Function1/1(s_act_lr), [s_act_lr]
  MATLAB Function1/1(flag_lr) -> [flag_lr], Scope1/1, Memory1/1
  Memory1/1 -> MATLAB Function1/4(flag_lr_pre)
  Constant1/1 -> MATLAB Function1/3(s_opt_zhuan_add)
  s_act_rf/1 -> [s_act_rf], MATLAB Function2/1(s_act_rf)
  MATLAB Function2/1(flag_rf) -> Memory2/1, [flag_rf], Scope2/1
  Memory2/1 -> MATLAB Function2/4(flag_rf_pre)
  Constant2/1 -> MATLAB Function2/3(s_opt_zhuan_add)
  s_act_rr/1 -> [s_act_rr], MATLAB Function3/1(s_act_rr)
  s_opt_zhuan/1 -> [s_opt_zhuan], MATLAB Function3/2(s_opt_zhuan), MATLAB Function2/2(s_opt_zhuan), MATLAB Function1/2(s_opt_zhuan), MATLAB Function/2(s_opt_zhuan)
  MATLAB Function3/1(flag_rr) -> [flag_rr], Scope3/1, Memory3/1
  Memory3/1 -> MATLAB Function3/4(flag_rr_pre)
  Constant3/1 -> MATLAB Function3/3(s_opt_zhuan_add)
  [flag_rf] -> MATLAB Function4/10(flag_rf)
  [flag_rr] -> MATLAB Function4/11(flag_rr)
  Mux/1 -> backward_dem/1

== system DDCU_wxt_v02_forA_LabviewV01/MainControl/mode_control/backward/backward/Drive/驱动防滑控制TCS/转向TCS/Subsystem ==
  speed_act_lf : Inport
  v_act : Inport  Port=2
  Add : Sum
  Constant : Constant  Value=eps
  Divide : Product  Inputs=*/
  Gain : Gain  Gain=pi/30
  Gain1 : Gain  Gain=Radius
  Gain2 : Gain  Gain=1/3.6
  Subtract : Sum  Inputs=+-
  s_act_lf : Outport
  wires:
  Divide/1 -> s_act_lf/1
  Add/1 -> Divide/2
  Constant/1 -> Add/2
  Subtract/1 -> Divide/1
  Gain2/1 -> Subtract/2
  Gain1/1 -> Subtract/1, Add/1
  v_act/1 -> Gain2/1
  Gain/1 -> Gain1/1
  speed_act_lf/1 -> Gain/1

== system DDCU_wxt_v02_forA_LabviewV01/MainControl/mode_control/backward/backward/Drive/驱动防滑控制TCS/转向TCS/Subsystem1 ==
  speed_act_lr : Inport
  v_act : Inport  Port=2
  Add : Sum
  Constant : Constant  Value=eps
  Divide : Product  Inputs=*/
  Gain : Gain  Gain=pi/30
  Gain1 : Gain  Gain=Radius
  Gain2 : Gain  Gain=1/3.6
  Subtract : Sum  Inputs=+-
  s_act_lr : Outport
  wires:
  speed_act_lr/1 -> Gain/1
  Gain/1 -> Gain1/1
  v_act/1 -> Gain2/1
  Gain1/1 -> Add/1, Subtract/1
  Gain2/1 -> Subtract/2
  Subtract/1 -> Divide/1
  Constant/1 -> Add/2
  Add/1 -> Divide/2
  Divide/1 -> s_act_lr/1

== system DDCU_wxt_v02_forA_LabviewV01/MainControl/mode_control/backward/backward/Drive/驱动防滑控制TCS/转向TCS/Subsystem2 ==
  speed_act_rf : Inport
  v_act : Inport  Port=2
  Add : Sum
  Constant : Constant  Value=eps
  Divide : Product  Inputs=*/
  Gain : Gain  Gain=pi/30
  Gain1 : Gain  Gain=Radius
  Gain2 : Gain  Gain=1/3.6
  Subtract : Sum  Inputs=+-
  s_act_rf : Outport
  wires:
  Divide/1 -> s_act_rf/1
  Add/1 -> Divide/2
  Constant/1 -> Add/2
  Subtract/1 -> Divide/1
  Gain2/1 -> Subtract/2
  Gain1/1 -> Subtract/1, Add/1
  v_act/1 -> Gain2/1
  Gain/1 -> Gain1/1
  speed_act_rf/1 -> Gain/1

== system DDCU_wxt_v02_forA_LabviewV01/MainControl/mode_control/backward/backward/Drive/驱动防滑控制TCS/转向TCS/Subsystem3 ==
  speed_act_rr : Inport
  v_act : Inport  Port=2
  Add : Sum
  Constant : Constant  Value=eps
  Divide : Product  Inputs=*/
  Gain : Gain  Gain=pi/30
  Gain1 : Gain  Gain=Radius
  Gain2 : Gain  Gain=1/3.6
  Subtract : Sum  Inputs=+-
  s_act_rr : Outport
  wires:
  speed_act_rr/1 -> Gain/1
  Gain/1 -> Gain1/1
  v_act/1 -> Gain2/1
  Gain1/1 -> Add/1, Subtract/1
  Gain2/1 -> Subtract/2
  Subtract/1 -> Divide/1
  Constant/1 -> Add/2
  Add/1 -> Divide/2
  Divide/1 -> s_act_rr/1

== matlab function DDCU_wxt_v02_forA_LabviewV01/MainControl/mode_control/forward/forward/Brake/HeartBeat ==
  data: life_pre input; life output
function life = fcn(life_pre)
%#codegen
life=life_pre+1;
if life>15
    life=0;
end
end

== matlab function DDCU_wxt_v02_forA_LabviewV01/MainControl/mode_control/neutral/neutral/HeartBeat1 ==
  data: life_pre input; life output
function life = fcn(life_pre)
%#codegen
life=life_pre+1;
if life>15
    life=0;
end
end

== matlab function DDCU_wxt_v02_forA_LabviewV01/MainControl/mode_control/center_steer/center_steer/HeartBeat ==
  data: life_pre input; life output
function life = fcn(life_pre)
%#codegen
life=life_pre+1;
if life>15
    life=0;
end
end

== matlab function DDCU_wxt_v02_forA_LabviewV01/MainControl/mode_control/center_steer/center_steer/HeartBeat1 ==
  data: life_pre input; life output
function life = fcn(life_pre)
%#codegen
life=life_pre+1;
if life>15
    life=0;
end
end

== matlab function DDCU_wxt_v02_forA_LabviewV01/MainControl/mode_control/forward/forward/Drive/驱动防滑控制TCS/直行TCS/直行/MATLAB Function2 ==
  data: s_act_rf input; flag_rf output; s_opt_zhuan input; s_opt_zhuan_add input; flag_rf_pre input
function flag_rf = fcn(s_act_rf,s_opt_zhuan,s_opt_zhuan_add,flag_rf_pre)
%#codegen
if s_act_rf>s_opt_zhuan+s_opt_zhuan_add
    flag_rf=1;
elseif s_act_rf<s_opt_zhuan
    flag_rf = 0;
else
    flag_rf=flag_rf_pre;
end
end

== matlab function DDCU_wxt_v02_forA_LabviewV01/InputSignalProcess/Subsystem/MATLAB Function ==
  data: zhuche input; mode_dem output; zhongxinzhuanxiang input; qianjin input; kongdang input; daodang input
function mode_dem = fcn(zhuche,zhongxinzhuanxiang,qianjin,kongdang,daodang)
%#codegen
if zhuche==1 && qianjin==0 && kongdang==0 && daodang==0 && zhongxinzhuanxiang==0
    mode_dem=0;     %驻车
elseif zhuche==0 && qianjin==1 && kongdang==0 && daodang==0 && zhongxinzhuanxiang==0
    mode_dem=1;  %前进
elseif zhuche==0 && qianjin==0 && kongdang==1 && daodang==0 && zhongxinzhuanxiang==0
    mode_dem=2;   %空挡
elseif zhuche==0 && qianjin==0 && kongdang==0 && daodang==1 && zhongxinzhuanxiang==0
    mode_dem=3; %倒车
elseif zhuche==0 && qianjin==0 && kongdang==0 && daodang==0 && zhongxinzhuanxiang==1
    mode_dem=4;%中心转向
else 
    mode_dem=5;%急停
end
end

== matlab function DDCU_wxt_v02_forA_LabviewV01/MainControl/mode_control/backward/backward/Drive/左右侧电机分配及功率限制/MATLAB Function ==
  data: trqlim_l input; trq_dem_l output; trq_dem_r output; trq_dem_l1 input; trqlim_r input; trq_dem_r1 input; delta_T_dem input
function [trq_dem_l,trq_dem_r] = fcn(trqlim_l,trq_dem_l1,trqlim_r,trq_dem_r1,delta_T_dem)
%#codegen
if trq_dem_l1==trqlim_l
    trq_dem_l=trq_dem_l1;
    trq_dem_r=trq_dem_l1+delta_T_dem;%这时候加的是负值
elseif trq_dem_r1==trqlim_r
    trq_dem_l=trq_dem_r1-delta_T_dem;
    trq_dem_r=trq_dem_r1;
    
else
    trq_dem_l=trq_dem_l1;
    trq_dem_r=trq_dem_r1;
end
% trq_dem_l=max(0,trq_dem_l);%限一下最小值，不要小于0
% trq_dem_r=max(0,trq_dem_r);
trq_dem_l=max(-trqlim_l,trq_dem_l);%小转向半径下，内侧履带是可能输出负转矩的，从地面吸收功率，给外侧，所以不能限到0，限到最大电机外特性负值
trq_dem_r=max(-trqlim_r,trq_dem_r);
end

== matlab function DDCU_wxt_v02_forA_LabviewV01/MainControl/mode_control/backward/backward/Drive/驱动防滑控制TCS/直行TCS/直行/MATLAB Function4 ==
  data: trq_dem_lf input; trq_dem_lr input; trq_dem_rf input; trq_dem_rr input; bra_pre_l input; bra_pre_r input; brakepre_dem input; flag_lf input; flag_lr input; trq_out_lf output; flag_rf input; flag_rr input; trq_out_lr output; trq_out_rf output; trq_out_rr output; trq_pid_lf input; trq_pid_lr input; trq_pid_rf input; trq_pid_rr input; brapre_out_l output; brapre_out_r output; mode output
function [trq_out_lf,trq_out_lr,trq_out_rf,trq_out_rr,brapre_out_l,brapre_out_r,mode] = fcn(trq_dem_lf,trq_dem_lr,trq_dem_rf,trq_dem_rr,bra_pre_l,bra_pre_r,brakepre_dem,flag_lf,flag_lr,flag_rf,flag_rr,trq_pid_lf,trq_pid_lr,trq_pid_rf,trq_pid_rr)
%#codegen pid模块在外面做，里面进行十六种情况的判断，先看一下效果，不能再修改。
if flag_lf==0 && flag_lr==0 && flag_rf==0 && flag_rr==0 % 0电机滑转===============================================0电机滑转
    trq_out_lf=trq_dem_lf;
    trq_out_lr=trq_dem_lr;
    trq_out_rf=trq_dem_rf;
    trq_out_rr=trq_dem_rr;
    brapre_out_l=bra_pre_l+brakepre_dem;
    brapre_out_r=bra_pre_r+brakepre_dem;
    mode=1;
elseif flag_lf==1 && flag_lr==0 &&flag_rf==0 && flag_rr==0 %左前轮滑转===================================================1电机滑转
    trq_out_lf=trq_pid_lf;
    trq_out_lr=trq_dem_lr+(trq_dem_lf-trq_out_lf);
    trq_out_rf=trq_dem_rf;
    trq_out_rr=trq_dem_rr;
    brapre_out_l=bra_pre_l+brakepre_dem;
    brapre_out_r=bra_pre_r+brakepre_dem;
    mode=2;
elseif flag_lf==0 && flag_lr==1 &&flag_rf==0 && flag_rr==0 %左后轮滑转
    trq_out_lr=trq_pid_lr;
    trq_out_lf=trq_dem_lf+(trq_dem_lr-trq_out_lr);
    trq_out_rf=trq_dem_rf;
    trq_out_rr=trq_dem_rr;
    brapre_out_l=bra_pre_l+brakepre_dem;
    brapre_out_r=bra_pre_r+brakepre_dem;
    mode=3;
elseif flag_lf==0 && flag_lr==0 &&flag_rf==1 && flag_rr==0 %右前轮滑转
    trq_out_rf=trq_pid_rf;
    trq_out_rr=trq_dem_rr+(trq_dem_rf-trq_out_rf);
    trq_out_lf=trq_dem_lf;
    trq_out_lr=trq_dem_lr;
    brapre_out_l=bra_pre_l+brakepre_dem;
    brapre_out_r=bra_pre_r+brakepre_dem;
    mode=4;
elseif flag_lf==0 && flag_lr==0 &&flag_rf==0 && flag_rr==1 %右后轮滑转
    trq_out_rr=trq_pid_rr;
    trq_out_rf=trq_dem_rf+(trq_dem_rr-trq_out_rr);
    trq_out_lf=trq_dem_lf;
    trq_out_lr=trq_dem_lr;
    brapre_out_l=bra_pre_l+brakepre_dem;
    brapre_out_r=bra_pre_r+brakepre_dem;
    mode=5;
elseif flag_lf==1 && flag_lr==1 &&flag_rf==0 && flag_rr==0 %左侧两轮滑转=====================================================================2电机滑转
    trq_out_lf=trq_pid_lf;
    trq_out_lr=trq_pid_lr;
    trq_out_rf=trq_dem_rf-(trq_dem_lf+trq_dem_lr-trq_out_lf-trq_out_lr)/2;
    trq_out_rr=trq_dem_rr-(trq_dem_lf+trq_dem_lr-trq_out_lf-trq_out_lr)/2;
    brapre_out_l=bra_pre_l+brakepre_dem;
    brapre_out_r=bra_pre_r+brakepre_dem;
    mode=6;
elseif flag_lf==0 && flag_lr==0 &&flag_rf==1 && flag_rr==1 %右侧两轮滑转
    trq_out_rf=trq_pid_rf;
    trq_out_rr=trq_pid_rr;
    trq_out_lf=trq_dem_lf-(trq_dem_rf+trq_dem_rr-trq_out_rf-trq_out_rr)/2;
    trq_out_lr=trq_dem_lr-(trq_dem_rf+trq_dem_rr-trq_out_rf-trq_out_rr)/2;
    brapre_out_l=bra_pre_l+brakepre_dem;
    brapre_out_r=bra_pre_r+brakepre_dem;
    mode=7;
elseif flag_lf==1 && flag_lr==0 &&flag_rf==1 && flag_rr==0 %前轴滑转
    trq_out_lf=trq_pid_lf;
    trq_out_lr=trq_dem_lr+(trq_dem_lf-trq_out_lf);
    trq_out_rf=trq_pid_rf;
    trq_out_rr=trq_dem_rr+(trq_dem_rf-trq_out_rf);
    brapre_out_l=bra_pre_l+brakepre_dem;
    brapre_out_r=bra_pre_r+brakepre_dem;
    mode=8;
elseif flag_lf==0 && flag_lr==1 &&flag_rf==0 && flag_rr==1 %后轴滑转
    trq_out_lr=trq_pid_lr;
    trq_out_lf=trq_dem_lf+(trq_dem_lr-trq_out_lr);
    trq_out_rr=trq_pid_rr;
    trq_out_rf=trq_dem_rf+(trq_dem_rr-trq_out_rr);
    brapre_out_l=bra_pre_l+brakepre_dem;
    brapre_out_r=bra_pre_r+brakepre_dem;
    mode=9;
elseif flag_lf==1 && flag_lr==0 &&flag_rf==0 && flag_rr==1 %左前轮和右后轮滑转
    trq_out_lf=trq_pid_lf;
    trq_out_lr=trq_dem_lr+(trq_dem_lf-trq_out_lf);
    trq_out_rr=trq_pid_rr;
    trq_out_rf=trq_dem_rf+(trq_dem_rr-trq_out_rr);
    brapre_out_l=bra_pre_l+brakepre_dem;
    brapre_out_r=bra_pre_r+brakepre_dem;
    mode=10;
elseif flag_lf==0 && flag_lr==1 &&flag_rf==1 && flag_rr==0 %左后轮和右前轮滑转
    trq_out_lr=trq_pid_lr;
    trq_out_lf=trq_dem_lf+(trq_dem_lr-trq_out_lr);
    trq_out_rf=trq_pid_rf;
    trq_out_rr=trq_dem_rr+(trq_dem_rf-trq_out_rf);
    brapre_out_l=bra_pre_l+brakepre_dem;
    brapre_out_r=bra_pre_r+brakepre_dem;
    mode=11;
elseif flag_lf==1 && flag_lr==1 &&flag_rf==1 && flag_rr==0 %右后不滑转======================================================================3电机滑转
    trq_out_lf=trq_pid_lf;
    trq_out_lr=trq_pid_lr;
    trq_out_rf=trq_pid_rf;
    trq_out_rr=trq_dem_rr+(trq_dem_rf-trq_out_rf)-(trq_dem_lf+trq_dem_lr-trq_out_lf-trq_out_lr);
    brapre_out_l=bra_pre_l+brakepre_dem;
    brapre_out_r=bra_pre_r+brakepre_dem;
    mode=12;
elseif flag_lf==1 && flag_lr==1 &&flag_rf==0 && flag_rr==1 %右前不滑转
    trq_out_lf=trq_pid_lf;
    trq_out_lr=trq_pid_lr;
    trq_out_rr=trq_pid_rr;
    trq_out_rf=trq_dem_rf+(trq_dem_rr-trq_out_rr)-(trq_dem_lf+trq_dem_lr-trq_out_lf-trq_out_lr);
    brapre_out_l=bra_pre_l+brakepre_dem;
    brapre_out_r=bra_pre_r+brakepre_dem;
    mode=13;
elseif flag_lf==1 && flag_lr==0 &&flag_rf==1 && flag_rr==1 %左后不滑转
    trq_out_rf=trq_pid_rf;
    trq_out_rr=trq_pid_rr;
    trq_out_lf=trq_pid_lf;
    trq_out_lr=trq_dem_lr+(trq_dem_lf-trq_out_lf)-(trq_dem_rf+trq_dem_rr-trq_out_rf-trq_out_rr);
    brapre_out_l=bra_pre_l+brakepre_dem;
    brapre_out_r=bra_pre_r+brakepre_dem;
    mode=14;
elseif flag_lf==0 && flag_lr==1 &&flag_rf==1 && flag_rr==1 %左前不滑转
    trq_out_rf=trq_pid_rf;
    trq_out_rr=trq_pid_rr;
    trq_out_lr=trq_pid_lr;
    trq_out_lf=trq_dem_lf+(trq_dem_lr-trq_out_lr)-(trq_dem_rf+trq_dem_rr-trq_out_rf-trq_out_rr);
    brapre_out_l=bra_pre_l+brakepre_dem;
    brapre_out_r=bra_pre_r+brakepre_dem;
    mode=15;
else
    %     flag_lf==1 && flag_lr==1 &&flag_rf==1 && flag_rr==1 %4电机均滑转======================================================================4电机均滑转
    trqcha=(trq_pid_lf+trq_pid_lr)-(trq_pid_rf+trq_pid_rr);
    if trqcha>0
        trq_out_rf=trq_pid_rf;
        trq_out_rr=trq_pid_rr;
        trq_out_lf=trq_pid_lf-(trq_pid_lf/(trq_pid_lf+trq_pid_lr))*trqcha;
        trq_out_lr=trq_pid_lr-(trq_pid_lr/(trq_pid_lf+trq_pid_lr))*trqcha;
    else
        trq_out_lf=trq_pid_lf;
        trq_out_lr=trq_pid_lr;
        trq_out_rf=trq_pid_rf+(trq_pid_rf/(trq_pid_rf+trq_pid_rr))*trqcha;
        trq_out_rr=trq_pid_rr+(trq_pid_rr/(trq_pid_rf+trq_pid_rr))*trqcha;
    end
    brapre_out_l=bra_pre_l+brakepre_dem;
    brapre_out_r=bra_pre_r+brakepre_dem;
    mode=16;
end
trq_out_lf=max(0,trq_out_lf);
trq_out_lr=max(0,trq_out_lr);
trq_out_rf=max(0,trq_out_rf);
trq_out_rr=max(0,trq_out_rr);
brapre_out_l=brapre_out_l;
brapre_out_r=brapre_out_r;
end
